simulink model "Copy_of_VTOLTiltrotor"  (R2024a)
settings: configuration reference "VTOLConfiguration" (kept outside this file)
undefined symbols (not defined in the file): airspeed, Battery, BCE12, BCE_Set_init, BMS_Controller_State, C, Cell10_P, Cell11_P, Cell12_P, Cell1_N, Cell1_P, Cell2_P, Cell3_P, Cell4_P, Cell5_P, Cell6_P, Cell7_P, Cell8_P, Cell9_P, Cell_Temperatures, Cell_Voltages, Charging_State, CityMission, control, controlParams, ControlSampleTime, CriticalTiltAngle, currentFactor, CV_Gain, ddx, ddy, ddz, Device_01, DiscIntNeverNeededParam, dx, dy, dz, Earth, env, F, F28379D_ADC_MaxCount, F28379D_ADC_Vmax, FixedWingMission, flightState, Foc_Ki_IxTcpu, Foc_Ki_S, Foc_Kp_I, Foc_Kp_S, fractalcoef, FSState, FWControlParams, HoverMission, I_cc, Ia_offset, Ib_offset, iniRoll, initPitch, iniYaw, IO334, IO334_DAC_Vmax ... (+55)
libraries: slrealtimeethercatlib x109, simulink x81, fl_lib x65, slpidlib x49, mcbcontrolslib x48, nesl_utility x43, speedgoatlib_hdlCoder_IO3xx x31, canmsglib x17, slrealtimeutilitieslib x13, mcbhdlplantlib x13, speedgoatlib_IO611 x12, dspstat3 x12
(part 12 of 20)

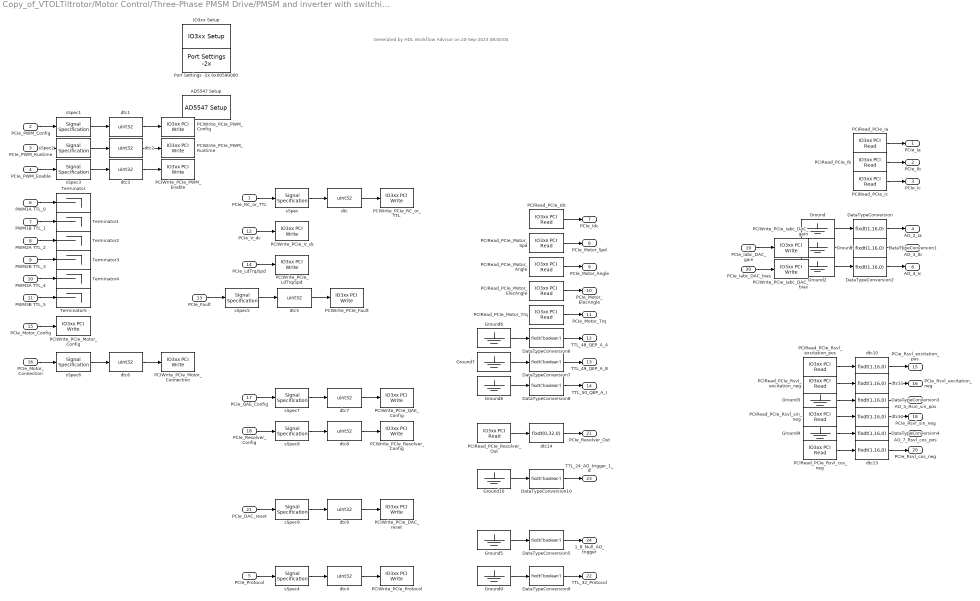
== system Copy_of_VTOLTiltrotor/Motor Control/Three-Phase PMSM Drive/PMSM and inverter with switching dynamics/PMSM_3P2L_Inverter_Plant_TBR/PMSM_3P2L_Inverter_Plant1 ==
  note: Generated by HDL Workflow Advisor on 20-Sep-2023 08:00:04
  PCIe_RC_or_TTL : Inport
  PCIe_PWM_Config : Inport  Port=2
  PCIe_PWM_Runtime : Inport  Port=3
  PCIe_PWM_Enable : Inport  Port=4
  PCIe_Protocol : Inport  Port=5
  PWM1A TTL_0 : Inport  Port=6
  PWM1B TTL_1 : Inport  Port=7
  PWM2A TTL_2 : Inport  Port=8
  PWM2B TTL_3 : Inport  Port=9
  PWM3A TTL_4 : Inport  Port=10
  PWM3B TTL_5 : Inport  Port=11
  PCIe_V_dc : Inport  Port=12
  PCIe_Fault : Inport  Port=13
  PCIe_LdTrq/Spd : Inport  Port=14
  PCIe_Motor_Config : Inport  Port=15
  PCIe_Motor_Connection : Inport  Port=16
  PCIe_QAE_Config : Inport  Port=17
  PCIe_Resolver_Config : Inport  Port=18
  PCIe_Iabc_DAC_gain : Inport  Port=19
  PCIe_Iabc_DAC_bias : Inport  Port=20
  PCIe_DAC_reset : Inport  Port=21
  AD5547 Setup : speedgoatlib_hdlCoder_IO3xx/AD5547 Setup  module_id=module_id  dacGain_1=10.0V  dacActiv_1=off  dacGain_2=2.5V  dacActiv_2=on  dacGain_3=2.5V  dacActiv_3=on  dacGain_4=2.5V  dacActiv_4=on  dacGain_5=2.5V  dacActiv_5=on  dacGain_6=10.0V  dacActiv_6=off  dacGain_7=2.5V  dacActiv_7=on  dacGain_8=10.0V  dacActiv_8=off  dacGain_9=10.0V  dacActiv_9=off  dacGain_10=10.0V  dacActiv_10=off  dacGain_11=10.0V  dacActiv_11=off  dacGain_12=10.0V  dacActiv_12=off  dacGain_13=10.0V  dacActiv_13=off  dacGain_14=10.0V  dacActiv_14=off  dacGain_15=10.0V  dacActiv_15=off  dacGain_16=10.0V  dacActiv_16=off
  DataTypeConversion{,1..4} (5 alike) : DataTypeConversion  OutDataTypeStr=fixdt(1,16,0)  ConvertRealWorld=Stored Integer (SI)  SaturateOnIntegerOverflow=off  RndMeth=Floor
  DataTypeConversion{5..10} (6 alike) : DataTypeConversion  OutDataTypeStr=fixdt('boolean')  ConvertRealWorld=Stored Integer (SI)  SaturateOnIntegerOverflow=off  RndMeth=Floor
  Ground{,1..10} (11 alike) : Ground
  IO3xx Setup : speedgoatlib_hdlCoder_IO3xx/IO3xx Setup  mdl_ss_name=PMSM3P2LInverterCHIL_RA/PMSM_3P2L_Inverter_Plant  board_type=IO334-325k  fpga_sync_mode=on  reset_mode=on  reset_mode_stop=on  device_id=1  module_id=module_id  pci_slot=slot  fpga_mat_file=c:\hdl_prj3\hdlsrc\PMSM3P2LInverterCHIL_RA\PMSM_3P2L_Inverter_Plant.mat  timestamp_mcs=09/19/23 21:42:55  timestamp=2309192041  tsreg=hex2dec('8')  bsf_file=PMSM_3P2L_Inverter_Plant_2309192041.mcs  mcs=0  init_reg_list=[]
  PCIRead_PCIe_Ia : speedgoatlib_hdlCoder_IO3xx/IO3xx PCI Read  device_id=1  module_id=module_id  board_type=IO334-325k  port_name=PCIe_Ia  port_offset=hex2dec('128')  port_type=single  port_dim=1  strobe=0  sample_time=ts
  PCIRead_PCIe_Ib : speedgoatlib_hdlCoder_IO3xx/IO3xx PCI Read  device_id=1  module_id=module_id  board_type=IO334-325k  port_name=PCIe_Ib  port_offset=hex2dec('12C')  port_type=single  port_dim=1  strobe=0  sample_time=ts
  PCIRead_PCIe_Ic : speedgoatlib_hdlCoder_IO3xx/IO3xx PCI Read  device_id=1  module_id=module_id  board_type=IO334-325k  port_name=PCIe_Ic  port_offset=hex2dec('130')  port_type=single  port_dim=1  strobe=0  sample_time=ts
  PCIRead_PCIe_Idc : speedgoatlib_hdlCoder_IO3xx/IO3xx PCI Read  device_id=1  module_id=module_id  board_type=IO334-325k  port_name=PCIe_Idc  port_offset=hex2dec('134')  port_type=single  port_dim=1  strobe=0  sample_time=ts
  PCIRead_PCIe_Motor_Angle : speedgoatlib_hdlCoder_IO3xx/IO3xx PCI Read  device_id=1  module_id=module_id  board_type=IO334-325k  port_name=PCIe_Motor_Angle  port_offset=hex2dec('13C')  port_type=single  port_dim=1  strobe=0  sample_time=ts
  PCIRead_PCIe_Motor_ElecAngle : speedgoatlib_hdlCoder_IO3xx/IO3xx PCI Read  device_id=1  module_id=module_id  board_type=IO334-325k  port_name=PCIe_Motor_ElecAngle  port_offset=hex2dec('184')  port_type=single  port_dim=1  strobe=0  sample_time=ts
  PCIRead_PCIe_Motor_Spd : speedgoatlib_hdlCoder_IO3xx/IO3xx PCI Read  device_id=1  module_id=module_id  board_type=IO334-325k  port_name=PCIe_Motor_Spd  port_offset=hex2dec('138')  port_type=single  port_dim=1  strobe=0  sample_time=ts
  PCIRead_PCIe_Motor_Trq : speedgoatlib_hdlCoder_IO3xx/IO3xx PCI Read  device_id=1  module_id=module_id  board_type=IO334-325k  port_name=PCIe_Motor_Trq  port_offset=hex2dec('188')  port_type=single  port_dim=1  strobe=0  sample_time=ts
  PCIRead_PCIe_Resolver_Out : speedgoatlib_hdlCoder_IO3xx/IO3xx PCI Read  device_id=1  module_id=module_id  board_type=IO334-325k  port_name=PCIe_Resolver_Out  port_offset=hex2dec('1D0')  port_type=uint32  port_dim=3  strobe=hex2dec('1E0')  sample_time=ts
  PCIRead_PCIe_Rsvl_cos_neg : speedgoatlib_hdlCoder_IO3xx/IO3xx PCI Read  device_id=1  module_id=module_id  board_type=IO334-325k  port_name=PCIe_Rsvl_cos_neg  port_offset=hex2dec('198')  port_type=uint32  port_dim=1  strobe=0  sample_time=ts
  PCIRead_PCIe_Rsvl_excitation_neg : speedgoatlib_hdlCoder_IO3xx/IO3xx PCI Read  device_id=1  module_id=module_id  board_type=IO334-325k  port_name=PCIe_Rsvl_excitation_neg  port_offset=hex2dec('190')  port_type=uint32  port_dim=1  strobe=0  sample_time=ts
  PCIRead_PCIe_Rsvl_excitation_pos : speedgoatlib_hdlCoder_IO3xx/IO3xx PCI Read  device_id=1  module_id=module_id  board_type=IO334-325k  port_name=PCIe_Rsvl_excitation_pos  port_offset=hex2dec('194')  port_type=uint32  port_dim=1  strobe=0  sample_time=ts
  PCIRead_PCIe_Rsvl_sin_neg : speedgoatlib_hdlCoder_IO3xx/IO3xx PCI Read  device_id=1  module_id=module_id  board_type=IO334-325k  port_name=PCIe_Rsvl_sin_neg  port_offset=hex2dec('18C')  port_type=uint32  port_dim=1  strobe=0  sample_time=ts
  PCIWrite_PCIe_DAC_reset : speedgoatlib_hdlCoder_IO3xx/IO3xx PCI Write  device_id=1  module_id=module_id  board_type=IO334-325k  port_name=PCIe_DAC_reset  port_offset=hex2dec('124')  port_type=uint32  port_dim=1  strobe=0  sample_time=ts
  PCIWrite_PCIe_Fault : speedgoatlib_hdlCoder_IO3xx/IO3xx PCI Write  device_id=1  module_id=module_id  board_type=IO334-325k  port_name=PCIe_Fault  port_offset=hex2dec('110')  port_type=uint32  port_dim=1  strobe=0  sample_time=ts
  PCIWrite_PCIe_Iabc_DAC_bias : speedgoatlib_hdlCoder_IO3xx/IO3xx PCI Write  device_id=1  module_id=module_id  board_type=IO334-325k  port_name=PCIe_Iabc_DAC_bias  port_offset=hex2dec('120')  port_type=single  port_dim=1  strobe=0  sample_time=ts
  PCIWrite_PCIe_Iabc_DAC_gain : speedgoatlib_hdlCoder_IO3xx/IO3xx PCI Write  device_id=1  module_id=module_id  board_type=IO334-325k  port_name=PCIe_Iabc_DAC_gain  port_offset=hex2dec('11C')  port_type=single  port_dim=1  strobe=0  sample_time=ts
  PCIWrite_PCIe_LdTrq/Spd : speedgoatlib_hdlCoder_IO3xx/IO3xx PCI Write  device_id=1  module_id=module_id  board_type=IO334-325k  port_name=PCIe_LdTrq//Spd  port_offset=hex2dec('114')  port_type=single  port_dim=1  strobe=0  sample_time=ts
  PCIWrite_PCIe_Motor_Config : speedgoatlib_hdlCoder_IO3xx/IO3xx PCI Write  device_id=1  module_id=module_id  board_type=IO334-325k  port_name=PCIe_Motor_Config  port_offset=hex2dec('340')  port_type=single  port_dim=9  strobe=hex2dec('380')  sample_time=ts
  PCIWrite_PCIe_Motor_Connection : speedgoatlib_hdlCoder_IO3xx/IO3xx PCI Write  device_id=1  module_id=module_id  board_type=IO334-325k  port_name=PCIe_Motor_Connection  port_offset=hex2dec('118')  port_type=uint32  port_dim=1  strobe=0  sample_time=ts
  PCIWrite_PCIe_PWM_Config : speedgoatlib_hdlCoder_IO3xx/IO3xx PCI Write  device_id=1  module_id=module_id  board_type=IO334-325k  port_name=PCIe_PWM_Config  port_offset=hex2dec('200')  port_type=uint32  port_dim=48  strobe=hex2dec('300')  sample_time=ts
  PCIWrite_PCIe_PWM_Enable : speedgoatlib_hdlCoder_IO3xx/IO3xx PCI Write  device_id=1  module_id=module_id  board_type=IO334-325k  port_name=PCIe_PWM_Enable  port_offset=hex2dec('104')  port_type=uint32  port_dim=1  strobe=0  sample_time=ts
  PCIWrite_PCIe_PWM_Runtime : speedgoatlib_hdlCoder_IO3xx/IO3xx PCI Write  device_id=1  module_id=module_id  board_type=IO334-325k  port_name=PCIe_PWM_Runtime  port_offset=hex2dec('140')  port_type=uint32  port_dim=15  strobe=hex2dec('180')  sample_time=ts
  PCIWrite_PCIe_Protocol : speedgoatlib_hdlCoder_IO3xx/IO3xx PCI Write  device_id=1  module_id=module_id  board_type=IO334-325k  port_name=PCIe_Protocol  port_offset=hex2dec('108')  port_type=uint32  port_dim=1  strobe=0  sample_time=ts
  PCIWrite_PCIe_QAE_Config : speedgoatlib_hdlCoder_IO3xx/IO3xx PCI Write  device_id=1  module_id=module_id  board_type=IO334-325k  port_name=PCIe_QAE_Config  port_offset=hex2dec('3C0')  port_type=uint32  port_dim=8  strobe=hex2dec('3E0')  sample_time=ts
  PCIWrite_PCIe_RC_or_TTL : speedgoatlib_hdlCoder_IO3xx/IO3xx PCI Write  device_id=1  module_id=module_id  board_type=IO334-325k  port_name=PCIe_RC_or_TTL  port_offset=hex2dec('100')  port_type=uint32  port_dim=1  strobe=0  sample_time=ts
  PCIWrite_PCIe_Resolver_Config : speedgoatlib_hdlCoder_IO3xx/IO3xx PCI Write  device_id=1  module_id=module_id  board_type=IO334-325k  port_name=PCIe_Resolver_Config  port_offset=hex2dec('480')  port_type=uint32  port_dim=17  strobe=hex2dec('500')  sample_time=ts
  PCIWrite_PCIe_V_dc : speedgoatlib_hdlCoder_IO3xx/IO3xx PCI Write  device_id=1  module_id=module_id  board_type=IO334-325k  port_name=PCIe_V_dc  port_offset=hex2dec('10C')  port_type=single  port_dim=1  strobe=0  sample_time=ts
  Port Settings -2x 0x00590000 : speedgoatlib_hdlCoder_IO3xx/Port Settings -2x  module_id=module_id  rearIO=-21  PullRPort0=pull-up 3.3V  VioPort0=3.3V  PullRPort1=pull-up 3.3V  VioPort1=3.3V  PullRPort2=pull-up 3.3V  VioPort2=3.3V  PullRPort3=pull-up 3.3V  VioPort3=3.3V  PullRPort4=pull-up 3.3V  VioPort4=3.3V  PullRPort5=pull-up 3.3V  VioPort5=3.3V  PullRPort6=pull-up 3.3V  VioPort6=3.3V  I2cAddrOffset=5832704  DutAddrOffset=120
  Terminator{,1..5} (6 alike) : Terminator
  dtc{,1..9} (10 alike) : DataTypeConversion  OutDataTypeStr=uint32  ConvertRealWorld=Stored Integer (SI)  SaturateOnIntegerOverflow=off
  dtc{10..13} (4 alike) : DataTypeConversion  OutDataTypeStr=fixdt(1,16,0)  ConvertRealWorld=Stored Integer (SI)  SaturateOnIntegerOverflow=off
  dtc14 : DataTypeConversion  OutDataTypeStr=fixdt(0,32,0)  ConvertRealWorld=Stored Integer (SI)  SaturateOnIntegerOverflow=off
  sSpec{,3..4,6} (4 alike) : SignalSpecification  OutDataTypeStr=fixdt('boolean')
  sSpec{1,5,7..8} (4 alike) : SignalSpecification  OutDataTypeStr=fixdt(0,32,0)
  sSpec2 : SignalSpecification  OutDataTypeStr=fixdt(0,24,0)
  sSpec9 : SignalSpecification  OutDataTypeStr=fixdt(0,16,0)
  PCIe_Ia : Outport
  PCIe_Ib : Outport  Port=2
  PCIe_Ic : Outport  Port=3
  AO_2_Ia : Outport  Port=4
  AO_3_Ib : Outport  Port=5
  AO_4_Ic : Outport  Port=6
  PCIe_Idc : Outport  Port=7
  PCIe_Motor_Spd : Outport  Port=8
  PCIe_Motor_Angle : Outport  Port=9
  PCIe_Motor_ElecAngle : Outport  Port=10
  PCIe_Motor_Trq : Outport  Port=11
  TTL_48_QEP_A_A : Outport  Port=12
  TTL_49_QEP_A_B : Outport  Port=13
  "TTL_50_QEP_A_I   " : Outport  Port=14
  PCIe_Rsvl_excitation_pos : Outport  Port=15
  PCIe_Rsvl_excitation_neg : Outport  Port=16
  AO_5_Rsvl_sin_pos : Outport  Port=17
  PCIe_Rsvl_sin_neg : Outport  Port=18
  AO_7_Rsvl_cos_pos : Outport  Port=19
  PCIe_Rsvl_cos_neg : Outport  Port=20
  PCIe_Resolver_Out : Outport  Port=21
  TTL_32_Protocol : Outport  Port=22
  TTL_24_AO_trigger_1_8 : Outport  Port=23
  1_8_Null_AO_trigger : Outport  Port=24
  wires:
  PCIe_RC_or_TTL/1 -> sSpec/1
  sSpec/1 -> dtc/1
  dtc/1 -> PCIWrite_PCIe_RC_or_TTL/1
  PCIe_PWM_Config/1 -> sSpec1/1
  sSpec1/1 -> dtc1/1
  dtc1/1 -> PCIWrite_PCIe_PWM_Config/1
  PCIe_PWM_Runtime/1 -> sSpec2/1
  sSpec2/1 -> dtc2/1
  dtc2/1 -> PCIWrite_PCIe_PWM_Runtime/1
  PCIe_PWM_Enable/1 -> sSpec3/1
  sSpec3/1 -> dtc3/1
  dtc3/1 -> PCIWrite_PCIe_PWM_Enable/1
  PCIe_Protocol/1 -> sSpec4/1
  sSpec4/1 -> dtc4/1
  dtc4/1 -> PCIWrite_PCIe_Protocol/1
  PCIe_V_dc/1 -> PCIWrite_PCIe_V_dc/1
  PCIe_Fault/1 -> sSpec5/1
  sSpec5/1 -> dtc5/1
  dtc5/1 -> PCIWrite_PCIe_Fault/1
  PCIe_LdTrq/Spd/1 -> PCIWrite_PCIe_LdTrq/Spd/1
  PCIe_Motor_Config/1 -> PCIWrite_PCIe_Motor_Config/1
  PCIe_Motor_Connection/1 -> sSpec6/1
  sSpec6/1 -> dtc6/1
  dtc6/1 -> PCIWrite_PCIe_Motor_Connection/1
  PCIe_QAE_Config/1 -> sSpec7/1
  sSpec7/1 -> dtc7/1
  dtc7/1 -> PCIWrite_PCIe_QAE_Config/1
  PCIe_Resolver_Config/1 -> sSpec8/1
  sSpec8/1 -> dtc8/1
  dtc8/1 -> PCIWrite_PCIe_Resolver_Config/1
  PCIe_Iabc_DAC_gain/1 -> PCIWrite_PCIe_Iabc_DAC_gain/1
  PCIe_Iabc_DAC_bias/1 -> PCIWrite_PCIe_Iabc_DAC_bias/1
  PCIe_DAC_reset/1 -> sSpec9/1
  sSpec9/1 -> dtc9/1
  dtc9/1 -> PCIWrite_PCIe_DAC_reset/1
  PCIRead_PCIe_Ia/1 -> PCIe_Ia/1
  PCIRead_PCIe_Ib/1 -> PCIe_Ib/1
  PCIRead_PCIe_Ic/1 -> PCIe_Ic/1
  PCIRead_PCIe_Idc/1 -> PCIe_Idc/1
  PCIRead_PCIe_Motor_Spd/1 -> PCIe_Motor_Spd/1
  PCIRead_PCIe_Motor_Angle/1 -> PCIe_Motor_Angle/1
  PCIRead_PCIe_Motor_ElecAngle/1 -> PCIe_Motor_ElecAngle/1
  PCIRead_PCIe_Motor_Trq/1 -> PCIe_Motor_Trq/1
  dtc10/1 -> PCIe_Rsvl_excitation_pos/1
  PCIRead_PCIe_Rsvl_excitation_pos/1 -> dtc10/1
  dtc11/1 -> PCIe_Rsvl_excitation_neg/1
  PCIRead_PCIe_Rsvl_excitation_neg/1 -> dtc11/1
  dtc12/1 -> PCIe_Rsvl_sin_neg/1
  PCIRead_PCIe_Rsvl_sin_neg/1 -> dtc12/1
  dtc13/1 -> PCIe_Rsvl_cos_neg/1
  PCIRead_PCIe_Rsvl_cos_neg/1 -> dtc13/1
  dtc14/1 -> PCIe_Resolver_Out/1
  PCIRead_PCIe_Resolver_Out/1 -> dtc14/1
  DataTypeConversion/1 -> AO_2_Ia/1
  Ground/1 -> DataTypeConversion/1
  DataTypeConversion1/1 -> AO_3_Ib/1
  Ground1/1 -> DataTypeConversion1/1
  DataTypeConversion2/1 -> AO_4_Ic/1
  Ground2/1 -> DataTypeConversion2/1
  DataTypeConversion3/1 -> AO_5_Rsvl_sin_pos/1
  Ground3/1 -> DataTypeConversion3/1
  DataTypeConversion4/1 -> AO_7_Rsvl_cos_pos/1
  Ground4/1 -> DataTypeConversion4/1
  DataTypeConversion5/1 -> 1_8_Null_AO_trigger/1
  Ground5/1 -> DataTypeConversion5/1
  PWM1A TTL_0/1 -> Terminator/1
  PWM1B TTL_1/1 -> Terminator1/1
  PWM2A TTL_2/1 -> Terminator2/1
  PWM2B TTL_3/1 -> Terminator3/1
  PWM3A TTL_4/1 -> Terminator4/1
  PWM3B TTL_5/1 -> Terminator5/1
  DataTypeConversion6/1 -> TTL_48_QEP_A_A/1
  Ground6/1 -> DataTypeConversion6/1
  DataTypeConversion7/1 -> TTL_49_QEP_A_B/1
  Ground7/1 -> DataTypeConversion7/1
  DataTypeConversion8/1 -> "TTL_50_QEP_A_I   "/1
  Ground8/1 -> DataTypeConversion8/1
  DataTypeConversion9/1 -> TTL_32_Protocol/1
  Ground9/1 -> DataTypeConversion9/1
  DataTypeConversion10/1 -> TTL_24_AO_trigger_1_8/1
  Ground10/1 -> DataTypeConversion10/1

== system Copy_of_VTOLTiltrotor/Motor Control/Three-Phase PMSM Drive1/PMSM and average inverter/Encoder Simulation/Get_PU  ==
  rad : Inport
  Constant2 : Constant  Value=2*pi  OutDataTypeStr=single  SampleTime=-1
  Get_PU : Gain  Gain=1/(2*pi)  RndMeth=Simplest  OutDataTypeStr=Inherit: Same as input
  Mod : Math  Operator=mod
  PU : Outport  VectorParamsAs1DForOutWhenUnconnected=off
  wires:
  Get_PU/1 -> PU/1
  Mod/1 -> Get_PU/1
  Constant2/1 -> Mod/2
  rad/1 -> Mod/1

== system Copy_of_VTOLTiltrotor/Motor Control/Three-Phase PMSM Drive1/PMSM and average inverter/Encoder Simulation/Wrap ==
  in : Inport
  Constant2 : Constant  OutDataTypeStr=single  SampleTime=-1
  Mod : Math  Operator=mod
  out : Outport  VectorParamsAs1DForOutWhenUnconnected=off
  wires:
  Mod/1 -> out/1
  Constant2/1 -> Mod/2
  in/1 -> Mod/1

== system Copy_of_VTOLTiltrotor/Motor Control/Three-Phase PMSM Drive1/PMSM and average inverter/Runtime to DC/To Dc A1 ==
  A_on : Inport
  A_off : Inport  Port=2
  Add : Sum
  Add Constant1 : Bias  Bias=1  SaturateOnIntegerOverflow=off
  Data Type Conversion3 : DataTypeConversion  OutDataTypeStr=double  SaturateOnIntegerOverflow=off  RndMeth=Floor
  Data Type Conversion5 : DataTypeConversion  OutDataTypeStr=double  SaturateOnIntegerOverflow=off  RndMeth=Floor
  Divide : Product  Inputs=*/
  Gain1 : Gain  Gain=-2
  Dc : Outport
  wires:
  Data Type Conversion5/1 -> Add/2
  Add Constant1/1 -> Dc/1
  Gain1/1 -> Add Constant1/1
  Add/1 -> Divide/2
  Data Type Conversion3/1 -> Add/1, Divide/1
  A_off/1 -> Data Type Conversion5/1
  Divide/1 -> Gain1/1
  A_on/1 -> Data Type Conversion3/1

== system Copy_of_VTOLTiltrotor/Motor Control/Three-Phase PMSM Drive1/PMSM and average inverter/Runtime to DC/To Dc A2 ==
  A_on : Inport
  A_off : Inport  Port=2
  Add : Sum
  Add Constant1 : Bias  Bias=1  SaturateOnIntegerOverflow=off
  Data Type Conversion3 : DataTypeConversion  OutDataTypeStr=double  SaturateOnIntegerOverflow=off  RndMeth=Floor
  Data Type Conversion5 : DataTypeConversion  OutDataTypeStr=double  SaturateOnIntegerOverflow=off  RndMeth=Floor
  Divide : Product  Inputs=*/
  Gain1 : Gain  Gain=-2
  Dc : Outport
  wires:
  A_on/1 -> Data Type Conversion3/1
  Divide/1 -> Gain1/1
  A_off/1 -> Data Type Conversion5/1
  Data Type Conversion3/1 -> Divide/1, Add/1
  Add/1 -> Divide/2
  Gain1/1 -> Add Constant1/1
  Add Constant1/1 -> Dc/1
  Data Type Conversion5/1 -> Add/2

== system Copy_of_VTOLTiltrotor/Motor Control/Three-Phase PMSM Drive1/PMSM and average inverter/Runtime to DC/To Dc A3 ==
  A_on : Inport
  A_off : Inport  Port=2
  Add : Sum
  Add Constant1 : Bias  Bias=1  SaturateOnIntegerOverflow=off
  Data Type Conversion3 : DataTypeConversion  OutDataTypeStr=double  SaturateOnIntegerOverflow=off  RndMeth=Floor
  Data Type Conversion5 : DataTypeConversion  OutDataTypeStr=double  SaturateOnIntegerOverflow=off  RndMeth=Floor
  Divide : Product  Inputs=*/
  Gain1 : Gain  Gain=-2
  Dc : Outport
  wires:
  Data Type Conversion5/1 -> Add/2
  Add Constant1/1 -> Dc/1
  Gain1/1 -> Add Constant1/1
  Add/1 -> Divide/2
  Data Type Conversion3/1 -> Add/1, Divide/1
  A_off/1 -> Data Type Conversion5/1
  Divide/1 -> Gain1/1
  A_on/1 -> Data Type Conversion3/1

== system Copy_of_VTOLTiltrotor/Motor Control/Three-Phase PMSM Drive2/PMSM and average inverter/Encoder Simulation/Get_PU  ==
  rad : Inport
  Constant2 : Constant  Value=2*pi  OutDataTypeStr=single  SampleTime=-1
  Get_PU : Gain  Gain=1/(2*pi)  RndMeth=Simplest  OutDataTypeStr=Inherit: Same as input
  Mod : Math  Operator=mod
  PU : Outport  VectorParamsAs1DForOutWhenUnconnected=off
  wires:
  Get_PU/1 -> PU/1
  Mod/1 -> Get_PU/1
  Constant2/1 -> Mod/2
  rad/1 -> Mod/1

== system Copy_of_VTOLTiltrotor/Motor Control/Three-Phase PMSM Drive2/PMSM and average inverter/Encoder Simulation/Wrap ==
  in : Inport
  Constant2 : Constant  OutDataTypeStr=single  SampleTime=-1
  Mod : Math  Operator=mod
  out : Outport  VectorParamsAs1DForOutWhenUnconnected=off
  wires:
  Mod/1 -> out/1
  Constant2/1 -> Mod/2
  in/1 -> Mod/1

== system Copy_of_VTOLTiltrotor/Motor Control/Three-Phase PMSM Drive2/PMSM and average inverter/Runtime to DC/To Dc A1 ==
  A_on : Inport
  A_off : Inport  Port=2
  Add : Sum
  Add Constant1 : Bias  Bias=1  SaturateOnIntegerOverflow=off
  Data Type Conversion3 : DataTypeConversion  OutDataTypeStr=double  SaturateOnIntegerOverflow=off  RndMeth=Floor
  Data Type Conversion5 : DataTypeConversion  OutDataTypeStr=double  SaturateOnIntegerOverflow=off  RndMeth=Floor
  Divide : Product  Inputs=*/
  Gain1 : Gain  Gain=-2
  Dc : Outport
  wires:
  Data Type Conversion5/1 -> Add/2
  Add Constant1/1 -> Dc/1
  Gain1/1 -> Add Constant1/1
  Add/1 -> Divide/2
  Data Type Conversion3/1 -> Add/1, Divide/1
  A_off/1 -> Data Type Conversion5/1
  Divide/1 -> Gain1/1
  A_on/1 -> Data Type Conversion3/1

== system Copy_of_VTOLTiltrotor/Motor Control/Three-Phase PMSM Drive2/PMSM and average inverter/Runtime to DC/To Dc A2 ==
  A_on : Inport
  A_off : Inport  Port=2
  Add : Sum
  Add Constant1 : Bias  Bias=1  SaturateOnIntegerOverflow=off
  Data Type Conversion3 : DataTypeConversion  OutDataTypeStr=double  SaturateOnIntegerOverflow=off  RndMeth=Floor
  Data Type Conversion5 : DataTypeConversion  OutDataTypeStr=double  SaturateOnIntegerOverflow=off  RndMeth=Floor
  Divide : Product  Inputs=*/
  Gain1 : Gain  Gain=-2
  Dc : Outport
  wires:
  A_on/1 -> Data Type Conversion3/1
  Divide/1 -> Gain1/1
  A_off/1 -> Data Type Conversion5/1
  Data Type Conversion3/1 -> Divide/1, Add/1
  Add/1 -> Divide/2
  Gain1/1 -> Add Constant1/1
  Add Constant1/1 -> Dc/1
  Data Type Conversion5/1 -> Add/2

== system Copy_of_VTOLTiltrotor/Motor Control/Three-Phase PMSM Drive2/PMSM and average inverter/Runtime to DC/To Dc A3 ==
  A_on : Inport
  A_off : Inport  Port=2
  Add : Sum
  Add Constant1 : Bias  Bias=1  SaturateOnIntegerOverflow=off
  Data Type Conversion3 : DataTypeConversion  OutDataTypeStr=double  SaturateOnIntegerOverflow=off  RndMeth=Floor
  Data Type Conversion5 : DataTypeConversion  OutDataTypeStr=double  SaturateOnIntegerOverflow=off  RndMeth=Floor
  Divide : Product  Inputs=*/
  Gain1 : Gain  Gain=-2
  Dc : Outport
  wires:
  Data Type Conversion5/1 -> Add/2
  Add Constant1/1 -> Dc/1
  Gain1/1 -> Add Constant1/1
  Add/1 -> Divide/2
  Data Type Conversion3/1 -> Add/1, Divide/1
  A_off/1 -> Data Type Conversion5/1
  Divide/1 -> Gain1/1
  A_on/1 -> Data Type Conversion3/1

== system Copy_of_VTOLTiltrotor/Motor Control/Three-Phase PMSM Drive3/PMSM and average inverter/Encoder Simulation/Get_PU  ==
  rad : Inport
  Constant2 : Constant  Value=2*pi  OutDataTypeStr=single  SampleTime=-1
  Get_PU : Gain  Gain=1/(2*pi)  RndMeth=Simplest  OutDataTypeStr=Inherit: Same as input
  Mod : Math  Operator=mod
  PU : Outport  VectorParamsAs1DForOutWhenUnconnected=off
  wires:
  Get_PU/1 -> PU/1
  Mod/1 -> Get_PU/1
  Constant2/1 -> Mod/2
  rad/1 -> Mod/1

== system Copy_of_VTOLTiltrotor/Motor Control/Three-Phase PMSM Drive3/PMSM and average inverter/Encoder Simulation/Wrap ==
  in : Inport
  Constant2 : Constant  OutDataTypeStr=single  SampleTime=-1
  Mod : Math  Operator=mod
  out : Outport  VectorParamsAs1DForOutWhenUnconnected=off
  wires:
  Mod/1 -> out/1
  Constant2/1 -> Mod/2
  in/1 -> Mod/1

== system Copy_of_VTOLTiltrotor/Motor Control/Three-Phase PMSM Drive3/PMSM and average inverter/Runtime to DC/To Dc A1 ==
  A_on : Inport
  A_off : Inport  Port=2
  Add : Sum
  Add Constant1 : Bias  Bias=1  SaturateOnIntegerOverflow=off
  Data Type Conversion3 : DataTypeConversion  OutDataTypeStr=double  SaturateOnIntegerOverflow=off  RndMeth=Floor
  Data Type Conversion5 : DataTypeConversion  OutDataTypeStr=double  SaturateOnIntegerOverflow=off  RndMeth=Floor
  Divide : Product  Inputs=*/
  Gain1 : Gain  Gain=-2
  Dc : Outport
  wires:
  Data Type Conversion5/1 -> Add/2
  Add Constant1/1 -> Dc/1
  Gain1/1 -> Add Constant1/1
  Add/1 -> Divide/2
  Data Type Conversion3/1 -> Add/1, Divide/1
  A_off/1 -> Data Type Conversion5/1
  Divide/1 -> Gain1/1
  A_on/1 -> Data Type Conversion3/1

== system Copy_of_VTOLTiltrotor/Motor Control/Three-Phase PMSM Drive3/PMSM and average inverter/Runtime to DC/To Dc A2 ==
  A_on : Inport
  A_off : Inport  Port=2
  Add : Sum
  Add Constant1 : Bias  Bias=1  SaturateOnIntegerOverflow=off
  Data Type Conversion3 : DataTypeConversion  OutDataTypeStr=double  SaturateOnIntegerOverflow=off  RndMeth=Floor
  Data Type Conversion5 : DataTypeConversion  OutDataTypeStr=double  SaturateOnIntegerOverflow=off  RndMeth=Floor
  Divide : Product  Inputs=*/
  Gain1 : Gain  Gain=-2
  Dc : Outport
  wires:
  A_on/1 -> Data Type Conversion3/1
  Divide/1 -> Gain1/1
  A_off/1 -> Data Type Conversion5/1
  Data Type Conversion3/1 -> Divide/1, Add/1
  Add/1 -> Divide/2
  Gain1/1 -> Add Constant1/1
  Add Constant1/1 -> Dc/1
  Data Type Conversion5/1 -> Add/2

== system Copy_of_VTOLTiltrotor/Motor Control/Three-Phase PMSM Drive3/PMSM and average inverter/Runtime to DC/To Dc A3 ==
  A_on : Inport
  A_off : Inport  Port=2
  Add : Sum
  Add Constant1 : Bias  Bias=1  SaturateOnIntegerOverflow=off
  Data Type Conversion3 : DataTypeConversion  OutDataTypeStr=double  SaturateOnIntegerOverflow=off  RndMeth=Floor
  Data Type Conversion5 : DataTypeConversion  OutDataTypeStr=double  SaturateOnIntegerOverflow=off  RndMeth=Floor
  Divide : Product  Inputs=*/
  Gain1 : Gain  Gain=-2
  Dc : Outport
  wires:
  Data Type Conversion5/1 -> Add/2
  Add Constant1/1 -> Dc/1
  Gain1/1 -> Add Constant1/1
  Add/1 -> Divide/2
  Data Type Conversion3/1 -> Add/1, Divide/1
  A_off/1 -> Data Type Conversion5/1
  Divide/1 -> Gain1/1
  A_on/1 -> Data Type Conversion3/1

== system Copy_of_VTOLTiltrotor/Battery Management System/BMS/HIL/Controller/PLANT-Rx/Messages ==
  ID_0x201 : Inport
  ID_0x202 : Inport  Port=2
  ID_0x501 : Inport  Port=3
  ID_0x502 : Inport  Port=4
  Balancing : simulink/Sources/Enumerated Constant  OutDataTypeStr=Enum: BMS_Controller_State  Value=BMS_Controller_State.BMS_Idle  SampleTime=-1
  Balancing1 : simulink/Sources/Enumerated Constant  OutDataTypeStr=Enum: Charging_State  Value=Charging_State.Init  SampleTime=-1
  Bus Creator : BusCreator  Inputs=5  OutDataTypeStr=Bus: Faults
  CAN Unpack : canmsglib/CAN Unpack  MsgList=(none)  MsgName=CAN Msg  MsgIDType=Standard (11-bit identifier)  MsgIdentifier=0x201  MsgLength=8  SignalInfo={ 'DischargeCurrentLimit_CAN', '0', '32', 'LE', 'single', 'Standard', '0', '1', '0', '-inf', '+inf'; 'ChargeCurrentLimit_CAN', '32', '32', 'LE', 'single', 'Standard', '0', '1', '0', '-Inf', 'Inf' }  IDPort=off  TimestampPort=on  ErrorPort=off  RemotePort=off  LengthPort=off  StatusPort=on  ApplyMinMax=off
      settings: LibrarySourceBlock=embeddedtargetslib/Host Communication/CAN Unpack
  CAN Unpack1 : canmsglib/CAN Unpack  MsgList=(none)  MsgName=CAN Msg  MsgIDType=Standard (11-bit identifier)  MsgIdentifier=0x202  MsgLength=4  SignalInfo={ 'ChargeCurrentReq', '0', '32', 'LE', 'single', 'Standard', '0', '1', '0', '-inf', '+inf' }  IDPort=off  TimestampPort=on  ErrorPort=off  RemotePort=off  LengthPort=off  StatusPort=on  ApplyMinMax=off
      settings: LibrarySourceBlock=embeddedtargetslib/Host Communication/CAN Unpack
  CAN Unpack2 : canmsglib/CAN Unpack  MsgList=(none)  MsgName=CAN Msg  MsgIDType=Standard (11-bit identifier)  MsgIdentifier=0x501  MsgLength=8  SignalInfo={ 'SOC_UKF', '0', '32', 'LE', 'single', 'Standard', '0', '1', '0', '-inf', '+inf'; 'SOC_EKF', '32', '32', 'LE', 'single', 'Standard', '0', '1', '0', '-Inf', 'Inf' }  IDPort=off  TimestampPort=on  ErrorPort=off  RemotePort=off  LengthPort=off  StatusPort=on  ApplyMinMax=off
      settings: LibrarySourceBlock=embeddedtargetslib/Host Communication/CAN Unpack
  CAN Unpack3 : canmsglib/CAN Unpack  MsgList=(none)  MsgName=CAN Msg  MsgIDType=Standard (11-bit identifier)  MsgIdentifier=0x502  MsgLength=7  SignalInfo={ 'SOC_CC', '0', '32', 'LE', 'single', 'Standard', '0', '1', '0', '-inf', '+inf'; 'Faults', '32', '8', 'LE', 'unsigned', 'Standard', '0', '1', '0', '-Inf', 'Inf'; 'BMS_State', '40', '8', 'LE', 'unsigned', 'Standard', '0', '1', '0', '-Inf', 'Inf'; 'Charging_State', '48', '8', 'LE', 'signed', 'Standard', '0', '1', '0', '-Inf', 'Inf' }  IDPort=off  TimestampPort=on  ErrorPort=off  RemotePort=off  LengthPort=off  StatusPort=on  ApplyMinMax=off
      settings: LibrarySourceBlock=embeddedtargetslib/Host Communication/CAN Unpack
  Charging : simulink/Sources/Enumerated Constant  OutDataTypeStr=Enum: BMS_Controller_State  Value=BMS_Controller_State.BMS_Driving  SampleTime=-1
  Charging1 : simulink/Sources/Enumerated Constant  OutDataTypeStr=Enum: Charging_State  Value=Charging_State.CC  SampleTime=-1
  Driving : simulink/Sources/Enumerated Constant  OutDataTypeStr=Enum: BMS_Controller_State  Value=BMS_Controller_State.BMS_Charging  SampleTime=-1
  Driving1 : simulink/Sources/Enumerated Constant  OutDataTypeStr=Enum: BMS_Controller_State  Value=BMS_Controller_State.BMS_Fault  SampleTime=-1
  Driving2 : simulink/Sources/Enumerated Constant  OutDataTypeStr=Enum: Charging_State  Value=Charging_State.CV  SampleTime=-1
  Faults_unpacking : slrealtimeutilitieslib/Bit Unpacking  SignExtend=on  MaskBitPatterns={[7:7] [6:6] [5:5] [4:4] [3:3] [2:2] [1:1] [0:0]}  MaskPackDataType=uint8  MaskPackDataSize=[1]  MaskUnpackDataTypes={'boolean', 'boolean', 'boolean', 'boolean', 'boolean', 'boolean', 'boolean', 'boolean'}  MaskUnpackDataSizes={[1] [1] [1] [1] [1] [1] [1] [1]}
  Gain : Gain  Gain=100
  Gain1 : Gain  Gain=100
  Gain2 : Gain  Gain=100
  Multiport Switch1 : MultiPortSwitch  DataPortOrder=Zero-based contiguous  zeroidx=on  SaturateOnIntegerOverflow=off  InputSameDT=off
  Multiport Switch2 : MultiPortSwitch  DataPortOrder=Zero-based contiguous  Inputs=4  zeroidx=on  SaturateOnIntegerOverflow=off  InputSameDT=off
  Mux1 : Mux  Inputs=3
  Terminator{,1..2,4..5,7,10,13..16} (11 alike) : Terminator
  Discharge_Current_Limit : Outport
  Charge_Current_Limit : Outport  Port=2
  Charge_Current_Req : Outport  Port=3
  SOC : Outport  Port=4
  BMS_Faults : Outport  Port=5
  BMS_State : Outport  Port=6
  Charging_State : Outport  Port=7
  wires:
  CAN Unpack1/2 -> Terminator2/1
  CAN Unpack/1 -> Discharge_Current_Limit/1  "Discharge_Current_Limit"
  CAN Unpack1/1 -> Charge_Current_Req/1  "Charge_Current_Req"
  CAN Unpack1/3 -> Terminator5/1
  CAN Unpack/2 -> Charge_Current_Limit/1  "Charge_Current_Limit"
  CAN Unpack/4 -> Terminator7/1
  CAN Unpack/3 -> Terminator4/1
  ID_0x201/1 -> CAN Unpack/1
  ID_0x202/1 -> CAN Unpack1/1
  CAN Unpack2/2 -> Gain1/1
  Bus Creator/1 -> BMS_Faults/1
  Faults_unpacking/5 -> Bus Creator/5  "UnderVolt"
  CAN Unpack3/5 -> Terminator10/1
  CAN Unpack3/3 -> Multiport Switch2/1
  CAN Unpack3/2 -> Faults_unpacking/1
  Faults_unpacking/4 -> Bus Creator/4  "OverVolt"
  Faults_unpacking/3 -> Bus Creator/3  "LowTemp"
  CAN Unpack2/1 -> Gain/1
  Faults_unpacking/1 -> Bus Creator/1  "OverCurrent"
  ID_0x501/1 -> CAN Unpack2/1
  Faults_unpacking/2 -> Bus Creator/2  "HighTemp"
  CAN Unpack2/3 -> Terminator/1  "Time_0x501"
  ID_0x502/1 -> CAN Unpack3/1
  Gain/1 -> Mux1/1  "SOC_UKF"
  Gain1/1 -> Mux1/2  "SOC_EKF"
  CAN Unpack3/1 -> Gain2/1
  CAN Unpack2/4 -> Terminator1/1  "Status_0x501"
  Faults_unpacking/6 -> Terminator13/1
  Faults_unpacking/7 -> Terminator14/1
  Faults_unpacking/8 -> Terminator15/1
  CAN Unpack3/6 -> Terminator16/1
  Gain2/1 -> Mux1/3  "SOC_CC"
  Mux1/1 -> SOC/1  "SOC"
  Charging/1 -> Multiport Switch2/3
  Balancing/1 -> Multiport Switch2/2
  Driving/1 -> Multiport Switch2/4
  Driving1/1 -> Multiport Switch2/5
  Charging1/1 -> Multiport Switch1/3
  Driving2/1 -> Multiport Switch1/4
  Balancing1/1 -> Multiport Switch1/2
  CAN Unpack3/4 -> Multiport Switch1/1
  Multiport Switch1/1 -> Charging_State/1
  Multiport Switch2/1 -> BMS_State/1

== system Copy_of_VTOLTiltrotor/Battery Management System/BMS/HIL/Controller/PLANT-Tx/12-Cell ==
  to_Controller : Inport
  to_Controller_SRE : Inport  Port=2
  Bus Selector : BusSelector  OutputSignals=Pack_Current,Cell_Temperatures
  CAN Pack2 : canmsglib/CAN Pack  MsgList=(none)  MsgName=CAN Msg  MsgIDType=Standard (11-bit identifier)  MsgIdentifier=0x407  MsgLength=8  Remote=off  ApplyMinMax=off  BusOutput=off  SignalInfo={ 'Cell_Temperatures_2', '0', '32', 'LE', 'single', 'Standard', '0', '1', '0', '-Inf', 'Inf'; 'Cell_Temperatures_1', '32', '32', 'LE', 'single', 'Standard', '0', '1', '0', '-Inf', 'Inf' }
      settings: LibrarySourceBlock=embeddedtargetslib/Host Communication/CAN Pack  DataFormat=manually specified signals
  CAN Pack3 : canmsglib/CAN Pack  MsgList=(none)  MsgName=CAN Msg  MsgIDType=Standard (11-bit identifier)  MsgIdentifier=0x404  MsgLength=8  Remote=off  ApplyMinMax=off  BusOutput=off  SignalInfo={ 'Cell_Temperatures_8', '0', '32', 'LE', 'single', 'Standard', '0', '1', '0', '-Inf', 'Inf'; 'Cell_Temperatures_7', '32', '32', 'LE', 'single', 'Standard', '0', '1', '0', '-Inf', 'Inf' }
      settings: LibrarySourceBlock=embeddedtargetslib/Host Communication/CAN Pack  DataFormat=manually specified signals
  CAN Pack4 : canmsglib/CAN Pack  MsgList=(none)  MsgName=CAN Msg  MsgIDType=Standard (11-bit identifier)  MsgIdentifier=0x401  MsgLength=5  Remote=off  ApplyMinMax=off  BusOutput=off  SignalInfo={ 'Pack_Current', '0', '32', 'LE', 'single', 'Standard', '0', '1', '0', '-Inf', 'Inf'; 'SRE', '32', '8', 'LE', 'unsigned', 'Standard', '0', '1', '0', '-Inf', 'Inf' }
      settings: LibrarySourceBlock=embeddedtargetslib/Host Communication/CAN Pack  DataFormat=manually specified signals
  CAN Pack5 : canmsglib/CAN Pack  MsgList=(none)  MsgName=CAN Msg  MsgIDType=Standard (11-bit identifier)  MsgIdentifier=0x405  MsgLength=8  Remote=off  ApplyMinMax=off  BusOutput=off  SignalInfo={ 'Cell_Temperatures_6', '0', '32', 'LE', 'single', 'Standard', '0', '1', '0', '-Inf', 'Inf'; 'Cell_Temperatures_5', '32', '32', 'LE', 'single', 'Standard', '0', '1', '0', '-Inf', 'Inf' }
      settings: LibrarySourceBlock=embeddedtargetslib/Host Communication/CAN Pack  DataFormat=manually specified signals
  CAN Pack6 : canmsglib/CAN Pack  MsgList=(none)  MsgName=CAN Msg  MsgIDType=Standard (11-bit identifier)  MsgIdentifier=0x402  MsgLength=8  Remote=off  ApplyMinMax=off  BusOutput=off  SignalInfo={ 'Cell_Temperatures_12', '0', '32', 'LE', 'single', 'Standard', '0', '1', '0', '-Inf', 'Inf'; 'Cell_Temperatures_11', '32', '32', 'LE', 'single', 'Standard', '0', '1', '0', '-Inf', 'Inf' }
      settings: LibrarySourceBlock=embeddedtargetslib/Host Communication/CAN Pack  DataFormat=manually specified signals
  CAN Pack7 : canmsglib/CAN Pack  MsgList=(none)  MsgName=CAN Msg  MsgIDType=Standard (11-bit identifier)  MsgIdentifier=0x403  MsgLength=8  Remote=off  ApplyMinMax=off  BusOutput=off  SignalInfo={ 'Cell_Temperatures_10', '0', '32', 'LE', 'single', 'Standard', '0', '1', '0', '-Inf', 'Inf'; 'Cell_Temperatures_9', '32', '32', 'LE', 'single', 'Standard', '0', '1', '0', '-Inf', 'Inf' }
      settings: LibrarySourceBlock=embeddedtargetslib/Host Communication/CAN Pack  DataFormat=manually specified signals
  CAN Pack8 : canmsglib/CAN Pack  MsgList=(none)  MsgName=CAN Msg  MsgIDType=Standard (11-bit identifier)  MsgIdentifier=0x406  MsgLength=8  Remote=off  ApplyMinMax=off  BusOutput=off  SignalInfo={ 'Cell_Temperatures_4', '0', '32', 'LE', 'single', 'Standard', '0', '1', '0', '-Inf', 'Inf'; 'Cell_Temperatures_3', '32', '32', 'LE', 'single', 'Standard', '0', '1', '0', '-Inf', 'Inf' }
      settings: LibrarySourceBlock=embeddedtargetslib/Host Communication/CAN Pack  DataFormat=manually specified signals
  CAN Write{,1..6} (7 alike) : speedgoatlib_IO611/Legacy/CAN/CAN Write  id=1  sampleTime=-1  portSelection=2  messageType=CAN  BusInput=off  enaStatusPort=off  protl=IO611  ptIdx=1  isFDMod=1
      settings: SourceProductName=IO611
  Demux1 : Demux  Outputs=12
  wires:
  to_Controller/1 -> Bus Selector/1
  Bus Selector/1 -> CAN Pack4/1  "<Pack_Current>"
  Bus Selector/2 -> Demux1/1  "<Cell_Temperatures>"
  Demux1/1 -> CAN Pack6/1
  Demux1/2 -> CAN Pack6/2
  Demux1/3 -> CAN Pack7/1
  Demux1/4 -> CAN Pack7/2
  Demux1/5 -> CAN Pack3/1
  Demux1/6 -> CAN Pack3/2
  CAN Pack4/1 -> CAN Write/1
  CAN Pack6/1 -> CAN Write1/1
  to_Controller_SRE/1 -> CAN Pack4/2
  CAN Pack7/1 -> CAN Write2/1
  CAN Pack3/1 -> CAN Write3/1
  CAN Pack2/1 -> CAN Write6/1
  CAN Pack5/1 -> CAN Write4/1
  CAN Pack8/1 -> CAN Write5/1
  Demux1/7 -> CAN Pack5/1
  Demux1/8 -> CAN Pack5/2
  Demux1/9 -> CAN Pack8/1
  Demux1/10 -> CAN Pack8/2
  Demux1/11 -> CAN Pack2/1
  Demux1/12 -> CAN Pack2/2

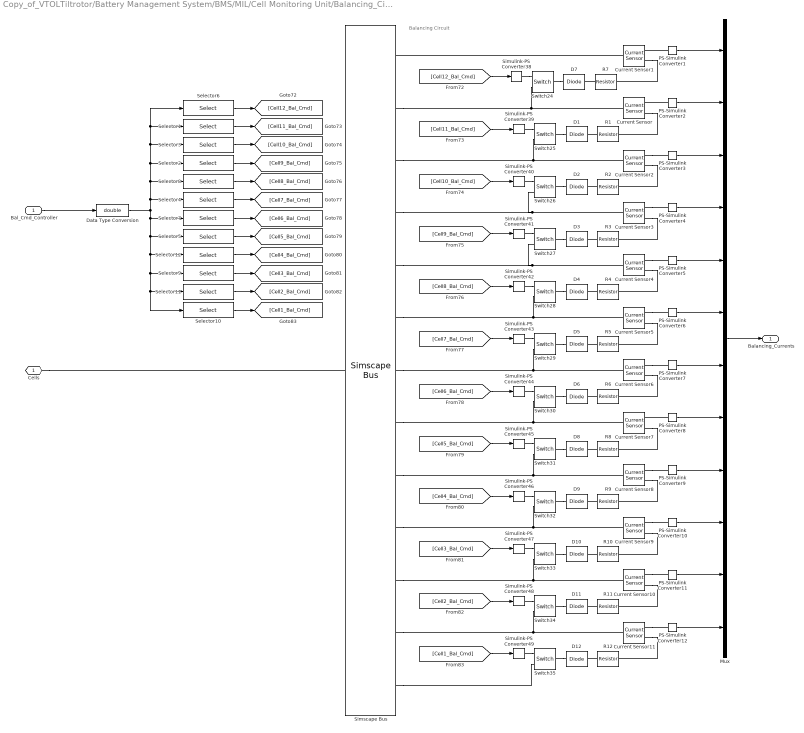
== system Copy_of_VTOLTiltrotor/Battery Management System/BMS/MIL/Cell Monitoring Unit/Balancing_Circuit/12-Cell ==
  note: Balancing Circuit
  Bal_Cmd_Controller : Inport
  Current Sensor{,1..11} (12 alike) : fl_lib/Electrical/Electrical Sensors/Current Sensor
  D{1..12} (12 alike) : fl_lib/Electrical/Electrical Elements/Diode  Vf=0.6 V  Ron=0.3 Ohm  Goff=1e-8 1/Ohm  i_specify=off  i_priority=High  i=0 A  i_nominal_specify=off  i_nominal_value=1  i_nominal_unit=A  v_specify=off  v_priority=None  v=0 V  v_nominal_specify=off  v_nominal_value=1  v_nominal_unit=V
      settings: LibrarySourceBlock=BatteryPack_lib/CellMonitoringUnit/D1  LogSimulationData=on
  Data Type Conversion : DataTypeConversion  OutDataTypeStr=double  SaturateOnIntegerOverflow=off  RndMeth=Floor
  Mux : Mux  Inputs=12
  PS-Simulink Converter{1..12} (12 alike) : nesl_utility/PS-Simulink Converter  PhysicalDomain=network_engine_domain  SubClassName=ps_output  LeftPortType=input  RightPortType=output  PseudoPeriodic=off  Frequencies=[]  VectorFormat=inherit  Unit=inherit  AffineConversion=off
  R{1..12} (12 alike) : fl_lib/Electrical/Electrical Elements/Resistor  R=Battery.R_bleed Ohm  i_specify=off  i_priority=None  i=0 A  i_nominal_specify=off  i_nominal_value=1  i_nominal_unit=A  v_specify=off  v_priority=None  v=0 V  v_nominal_specify=off  v_nominal_value=1  v_nominal_unit=V
      settings: LibrarySourceBlock=BatteryPack_lib/CellMonitoringUnit/R1  LogSimulationData=on
  Selector1 : Selector  IndexOptions=Index vector (dialog)  Indices=2  OutputSizes=1
  Selector10 : Selector  IndexOptions=Index vector (dialog)  Indices=12  OutputSizes=1
  Selector11 : Selector  IndexOptions=Index vector (dialog)  Indices=11  OutputSizes=1
  Selector12 : Selector  IndexOptions=Index vector (dialog)  Indices=9  OutputSizes=1
  Selector2 : Selector  IndexOptions=Index vector (dialog)  Indices=4  OutputSizes=1
  Selector3 : Selector  IndexOptions=Index vector (dialog)  Indices=3  OutputSizes=1
  Selector4 : Selector  IndexOptions=Index vector (dialog)  Indices=6  OutputSizes=1
  Selector5 : Selector  IndexOptions=Index vector (dialog)  Indices=8  OutputSizes=1
  Selector6 : Selector  IndexOptions=Index vector (dialog)  Indices=1  OutputSizes=1
  Selector7 : Selector  IndexOptions=Index vector (dialog)  Indices=7  OutputSizes=1
  Selector8 : Selector  IndexOptions=Index vector (dialog)  Indices=5  OutputSizes=1
  Selector9 : Selector  IndexOptions=Index vector (dialog)  Indices=10  OutputSizes=1
  Simscape Bus : SimscapeBus  HierarchyStrings=Cell12_P;Cell11_P;Cell10_P;Cell9_P;Cell8_P;Cell7_P;Cell6_P;Cell5_P;Cell4_P;Cell3_P;Cell2_P;Cell1_P;Cell1_N
  Simulink-PS Converter{38..49} (12 alike) : nesl_utility/Simulink-PS Converter  PhysicalDomain=network_engine_domain  SubClassName=ps_input  LeftPortType=input  RightPortType=output  PseudoPeriodic=off  Frequencies=[]  NoiseDistribution=none  NoiseParameters=[]  Unit=1  AffineConversion=off  FilteringAndDerivatives=zero  SimscapeFilterOrder=1  InputFilterTimeConstant=0.001  UdotUserProvided=1
      settings: LibrarySourceBlock=|
      | BatteryPack_lib/CellMonitoringUnit/Simulink-PS
      | Converter3
  Switch{24..35} (12 alike) : fl_lib/Electrical/Electrical Elements/Switch  R_closed=0.01 Ohm  G_open=1e-8 1/Ohm  Threshold=0  i_specify=off  i_priority=None  i=0 A  i_nominal_specify=off  i_nominal_value=1  i_nominal_unit=A  v_specify=off  v_priority=None  v=0 V  v_nominal_specify=off  v_nominal_value=1  v_nominal_unit=V
      settings: LibrarySourceBlock=BatteryPack_lib/CellMonitoringUnit/Switch
  Cells : PMIOPort  Side=Left
  Balancing_Currents : Outport
  wires:
  [Cell3_Bal_Cmd] -> Simulink-PS Converter47/1
  [Cell4_Bal_Cmd] -> Simulink-PS Converter46/1
  [Cell2_Bal_Cmd] -> Simulink-PS Converter48/1
  [Cell9_Bal_Cmd] -> Simulink-PS Converter41/1
  [Cell12_Bal_Cmd] -> Simulink-PS Converter38/1
  [Cell6_Bal_Cmd] -> Simulink-PS Converter44/1
  [Cell11_Bal_Cmd] -> Simulink-PS Converter39/1
  [Cell1_Bal_Cmd] -> Simulink-PS Converter49/1
  [Cell10_Bal_Cmd] -> Simulink-PS Converter40/1
  [Cell8_Bal_Cmd] -> Simulink-PS Converter42/1
  [Cell7_Bal_Cmd] -> Simulink-PS Converter43/1
  [Cell5_Bal_Cmd] -> Simulink-PS Converter45/1
  Selector11/1 -> [Cell2_Bal_Cmd]
  Selector12/1 -> [Cell4_Bal_Cmd]
  Selector3/1 -> [Cell10_Bal_Cmd]
  Selector9/1 -> [Cell3_Bal_Cmd]
  Selector1/1 -> [Cell11_Bal_Cmd]
  Selector4/1 -> [Cell7_Bal_Cmd]
  Selector8/1 -> [Cell8_Bal_Cmd]
  Selector6/1 -> [Cell12_Bal_Cmd]
  Selector7/1 -> [Cell6_Bal_Cmd]
  Selector5/1 -> [Cell5_Bal_Cmd]
  Selector10/1 -> [Cell1_Bal_Cmd]
  Selector2/1 -> [Cell9_Bal_Cmd]
  Data Type Conversion/1 -> Selector4/1, Selector8/1, Selector2/1, Selector3/1, Selector1/1, Selector6/1, Selector7/1, Selector5/1, Selector12/1, Selector9/1, Selector11/1, Selector10/1
  Bal_Cmd_Controller/1 -> Data Type Conversion/1
  PS-Simulink Converter1/1 -> Mux/1
  PS-Simulink Converter12/1 -> Mux/12
  PS-Simulink Converter2/1 -> Mux/2
  PS-Simulink Converter3/1 -> Mux/3
  PS-Simulink Converter4/1 -> Mux/4
  PS-Simulink Converter5/1 -> Mux/5
  PS-Simulink Converter6/1 -> Mux/6
  PS-Simulink Converter7/1 -> Mux/7
  PS-Simulink Converter8/1 -> Mux/8
  PS-Simulink Converter9/1 -> Mux/9
  PS-Simulink Converter10/1 -> Mux/10
  PS-Simulink Converter11/1 -> Mux/11
  Mux/1 -> Balancing_Currents/1
  connections:
  Simscape Bus/LConn6 -- Current Sensor5/LConn1 -- Switch28/RConn2
  Simscape Bus/LConn3 -- Current Sensor2/LConn1 -- Switch25/RConn2
  Simscape Bus/LConn5 -- Current Sensor4/LConn1 -- Switch27/RConn2
  Simscape Bus/LConn12 -- Current Sensor11/LConn1 -- Switch34/RConn2
  Simscape Bus/LConn4 -- Current Sensor3/LConn1 -- Switch26/RConn2
  Simscape Bus/LConn10 -- Current Sensor9/LConn1 -- Switch32/RConn2
  Simscape Bus/LConn8 -- Current Sensor7/LConn1 -- Switch30/RConn2
  Simscape Bus/LConn2 -- Current Sensor/LConn1 -- Switch24/RConn2
  Simscape Bus/LConn9 -- Current Sensor8/LConn1 -- Switch31/RConn2
  Simscape Bus/LConn7 -- Current Sensor6/LConn1 -- Switch29/RConn2
  Simscape Bus/LConn11 -- Current Sensor10/LConn1 -- Switch33/RConn2
  Simulink-PS Converter38/RConn1 -- Switch24/RConn1
  R4/RConn1 -- D4/LConn1
  Simulink-PS Converter48/RConn1 -- Switch34/RConn1
  R7/RConn1 -- D7/LConn1
  R8/RConn1 -- D8/LConn1
  Switch25/LConn1 -- D1/RConn1
  R6/RConn1 -- D6/LConn1
  R10/RConn1 -- D10/LConn1
  R12/RConn1 -- D12/LConn1
  Simulink-PS Converter49/RConn1 -- Switch35/RConn1
  R11/RConn1 -- D11/LConn1
  Switch30/LConn1 -- D6/RConn1
  Simulink-PS Converter41/RConn1 -- Switch27/RConn1
  Switch32/LConn1 -- D9/RConn1
  Switch31/LConn1 -- D8/RConn1
  Simulink-PS Converter39/RConn1 -- Switch25/RConn1
  Switch24/LConn1 -- D7/RConn1
  Simulink-PS Converter47/RConn1 -- Switch33/RConn1
  Simulink-PS Converter46/RConn1 -- Switch32/RConn1
  Switch35/LConn1 -- D12/RConn1
  Switch29/LConn1 -- D5/RConn1
  R2/RConn1 -- D2/LConn1
  Simulink-PS Converter44/RConn1 -- Switch30/RConn1
  Switch27/LConn1 -- D3/RConn1
  Switch28/LConn1 -- D4/RConn1
  Simulink-PS Converter43/RConn1 -- Switch29/RConn1
  Simulink-PS Converter45/RConn1 -- Switch31/RConn1
  R3/RConn1 -- D3/LConn1
  R9/RConn1 -- D9/LConn1
  Simulink-PS Converter42/RConn1 -- Switch28/RConn1
  Switch26/LConn1 -- D2/RConn1
  Simulink-PS Converter40/RConn1 -- Switch26/RConn1
  R5/RConn1 -- D5/LConn1
  Switch33/LConn1 -- D10/RConn1
  Switch34/LConn1 -- D11/RConn1
  R1/RConn1 -- D1/LConn1
  Simscape Bus/LConn13 -- Switch35/RConn2
  Cells/RConn1 -- Simscape Bus/RConn1
  Current Sensor1/LConn1 -- Simscape Bus/LConn1
  Current Sensor1/RConn2 -- R7/LConn1
  Current Sensor2/RConn2 -- R2/LConn1
  Current Sensor3/RConn2 -- R3/LConn1
  Current Sensor4/RConn2 -- R4/LConn1
  Current Sensor5/RConn2 -- R5/LConn1
  Current Sensor6/RConn2 -- R6/LConn1
  Current Sensor7/RConn2 -- R8/LConn1
  Current Sensor8/RConn2 -- R9/LConn1
  Current Sensor9/RConn2 -- R10/LConn1
  Current Sensor10/RConn2 -- R11/LConn1
  Current Sensor11/RConn2 -- R12/LConn1
  Current Sensor/RConn2 -- R1/LConn1
  PS-Simulink Converter1/LConn1 -- Current Sensor1/RConn1
  PS-Simulink Converter2/LConn1 -- Current Sensor/RConn1
  Current Sensor2/RConn1 -- PS-Simulink Converter3/LConn1
  Current Sensor3/RConn1 -- PS-Simulink Converter4/LConn1
  PS-Simulink Converter8/LConn1 -- Current Sensor7/RConn1
  Current Sensor6/RConn1 -- PS-Simulink Converter7/LConn1
  Current Sensor5/RConn1 -- PS-Simulink Converter6/LConn1
  Current Sensor4/RConn1 -- PS-Simulink Converter5/LConn1
  Current Sensor8/RConn1 -- PS-Simulink Converter9/LConn1
  Current Sensor9/RConn1 -- PS-Simulink Converter10/LConn1
  Current Sensor10/RConn1 -- PS-Simulink Converter11/LConn1
  Current Sensor11/RConn1 -- PS-Simulink Converter12/LConn1

== system Copy_of_VTOLTiltrotor/Battery Management System/BMS/MIL/Controller/Current Calculations/Charge_Current_Limit_Calc ==
  MaxCellVolt : Inport
  MinCellTemp : Inport  Port=2
  MaxCellTemp : Inport  Port=3
  Divide1 : Product  Inputs=*/
  HighTempChrgCurrentLim : Lookup_n-D  NumberOfTableDimensions=1  BreakpointsForDimension1=273.15+[-30:1:70]  Table=50*(1-tanh(273.15+[-30:1:70]-273.15-50))/2  InternalRulePriority=Speed  RndMeth=Simplest
  InternalCellResistance : Constant  Value=single(max(max(Battery(1).R0_LUT)))  OutDataTypeStr=single  SampleTime=-1
  LowTempChrgCurrentLim : Lookup_n-D  NumberOfTableDimensions=1  BreakpointsForDimension1=273.15+[-30:1:70]  Table=50*(1+tanh(273.15+[-30:1:70]-(273.15)))/2  InternalRulePriority=Speed  RndMeth=Simplest
  MinMax2 : MinMax  Inputs=3
  OverVoltageLimit : Constant  Value=OverCellVoltageLimit  OutDataTypeStr=single  SampleTime=-1
  Subtract1 : Sum  Inputs=+-
  Charge_Current_Limit : Outport  VectorParamsAs1DForOutWhenUnconnected=off
  wires:
  OverVoltageLimit/1 -> Subtract1/1
  MinMax2/1 -> Charge_Current_Limit/1  "ChargeCurrentLimit"
  MaxCellVolt/1 -> Subtract1/2
  Subtract1/1 -> Divide1/1
  Divide1/1 -> MinMax2/1
  InternalCellResistance/1 -> Divide1/2
  MinCellTemp/1 -> LowTempChrgCurrentLim/1
  MaxCellTemp/1 -> HighTempChrgCurrentLim/1
  HighTempChrgCurrentLim/1 -> MinMax2/3
  LowTempChrgCurrentLim/1 -> MinMax2/2

== system Copy_of_VTOLTiltrotor/Battery Management System/BMS/MIL/Controller/Current Calculations/Discharge_Current_Limit_Calc ==
  MinCellVolt : Inport
  MinCellTemp : Inport  Port=2
  MaxCellTemp : Inport  Port=3
  Divide : Product  Inputs=*/
  Gain : Gain  Gain=-1
  HighTempDchrgCurrentLim : Lookup_n-D  NumberOfTableDimensions=1  BreakpointsForDimension1=273.15+[-30:1:70]  Table=100*(1-tanh(273.15+[-30:1:70]-273.15-50))/2  InternalRulePriority=Speed  RndMeth=Simplest
  InternalCellResistance : Constant  Value=single(max(max(Battery(1).R0_LUT)))  OutDataTypeStr=single  SampleTime=-1
  LowTempDchrgCurrentLim : Lookup_n-D  NumberOfTableDimensions=1  BreakpointsForDimension1=273.15+[-30:1:70]  Table=100*(1+tanh(273.15+[-30:1:70]-(273.15)))/2  InternalRulePriority=Speed  RndMeth=Simplest
  MinMax2 : MinMax  Inputs=3
  Subtract : Sum  Inputs=+-
  UnderVoltageLimit : Constant  Value=UnderCellVoltageLimit  OutDataTypeStr=single  SampleTime=-1
  Discharge_Current_Limit : Outport  VectorParamsAs1DForOutWhenUnconnected=off
  wires:
  MinMax2/1 -> Gain/1  "DischargeCurrentLimit"
  Divide/1 -> MinMax2/1
  MinCellVolt/1 -> Subtract/1
  InternalCellResistance/1 -> Divide/2
  Subtract/1 -> Divide/1
  UnderVoltageLimit/1 -> Subtract/2
  Gain/1 -> Discharge_Current_Limit/1
  MaxCellTemp/1 -> HighTempDchrgCurrentLim/1
  MinCellTemp/1 -> LowTempDchrgCurrentLim/1
  HighTempDchrgCurrentLim/1 -> MinMax2/3
  LowTempDchrgCurrentLim/1 -> MinMax2/2

== system Copy_of_VTOLTiltrotor/Battery Management System/BMS/MIL/Controller/SOC Calculation/Coulomb Counting ==
  Curr : Inport
  Temp : Inport  Port=2
  1-D Lookup Table : Lookup_n-D  NumberOfTableDimensions=1  BreakpointsForDimension1=single(Battery(1).Temperature_LUT)  Table=single(Battery(1).Capacity_LUT)  InternalRulePriority=Speed  RndMeth=Simplest
  Discrete-Time Integrator : DiscreteIntegrator  InitialCondition=single(SOCInit+0.05)  SampleTime=-1  LimitOutput=on  UpperSaturationLimit=1  LowerSaturationLimit=0  ICPrevOutput=DiscIntNeverNeededParam  ICPrevScaledInput=DiscIntNeverNeededParam
  Divide : Product  Inputs=*/
  Gain : Gain  Gain=single(1/3600)
  SOC : Outport  VectorParamsAs1DForOutWhenUnconnected=off
  wires:
  Discrete-Time Integrator/1 -> SOC/1
  Curr/1 -> Gain/1
  Gain/1 -> Divide/1
  Divide/1 -> Discrete-Time Integrator/1
  1-D Lookup Table/1 -> Divide/2  "Capacity"
  Temp/1 -> 1-D Lookup Table/1

== system Copy_of_VTOLTiltrotor/Battery Management System/BMS/MIL/Controller/SOC Calculation/Measurement Function ==
  Current : Inport
  Temperature (K) : Inport  Port=2
  batteryMeasurementFcn : TriggerPort  TriggerType=function-call  IsSimulinkFunction=on  FunctionName=batteryMeasurementFcn  VariantControl=Variant
  Add1 : Sum  Inputs=+--
  Em Table : Lookup_n-D  BreakpointsForDimension1=Battery.SOC_LUT  BreakpointsForDimension2=Battery.Temperature_LUT  BeginIndexSearchUsingPreviousIndexResult=on  Table=Battery.Em_LUT  ExtrapMethod=Clip  InternalRulePriority=Speed  RndMeth=Simplest
      settings: InputPortMap=u0,u1
  Get SOC : Selector  InputPortWidth=2  IndexOptions=Index vector (dialog)  Indices=[1]  OutputSizes=1
  Get U1 : Selector  InputPortWidth=2  IndexOptions=Index vector (dialog)  Indices=2  OutputSizes=1
  Product : Product
  R0 Table : Lookup_n-D  BreakpointsForDimension1=Battery.SOC_LUT  BreakpointsForDimension2=Battery.Temperature_LUT  BeginIndexSearchUsingPreviousIndexResult=on  Table=Battery.R0_LUT  ExtrapMethod=Clip  InternalRulePriority=Speed  RndMeth=Simplest
      settings: InputPortMap=u0,u1
  x : ArgIn  DisableCoverage=on  OutDataTypeStr=single  PortDimensions=2  ArgumentName=x
  y : ArgOut  DisableCoverage=on  OutDataTypeStr=single  ArgumentName=y
  wires:
  Get U1/1 -> Add1/3  "U1"
  Product/1 -> Add1/2
  Current/1 -> Product/2
  R0 Table/1 -> Product/1
  Temperature (K)/1 -> Em Table/2, R0 Table/2
  Add1/1 -> y/1
  Em Table/1 -> Add1/1
  Get SOC/1 -> Em Table/1, R0 Table/1  "SOC"
  x/1 -> Get SOC/1, Get U1/1
